simulink model "lookupTableDynamic_TestGen14"  (R2017b)
settings: Solver=FixedStepDiscrete  StartTime=0.0  StopTime=10.0  RelTol=1e-3
libraries: simulink x1
settings Model: Creator=ktrinh  LastModifiedBy=ktrinh
settings DebuggingCC: ParameterOverflowMsg=none

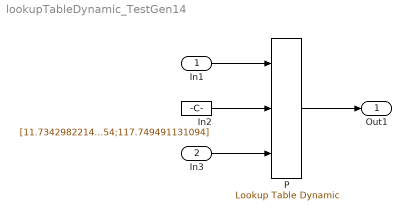
== system lookupTableDynamic_TestGen14 ==
  In1 : Inport  OutMin=9.7343  OutMax=120  OutDataTypeStr=uint16  PortDimensions=3
  In3 : Inport  Port=2  PortDimensions=5
  In2 : Constant  Value=[11.7342982214249;51.3502358259451;56.2803469538739;105.346904207054;117.749491131094]  OutDataTypeStr=uint16
  P : simulink/Lookup Tables/Lookup Table Dynamic  LookUpMeth=Interpolation-Use End Values  OutDataType=fixdt('int16')  OutScaling=[]  OutputDataTypeScalingMode=Specify via dialog  OutDataTypeStr=int16  RndMeth=Ceiling  DoSatur=off
      settings: SourceProductName=Simulink
  Out1 : Outport
  wires:
  In1/1 -> P/1
  In2/1 -> P/2
  In3/1 -> P/3
  P/1 -> Out1/1
